simulink model "SS_task9_2021"  (R2021b)
settings: Solver=FixedStepAuto  StartTime=0.0  StopTime=20  FixedStep=0.01  RelTol=1e-3
values from neighbouring files (symbols this model uses):
  A_ss_2dof_vh = eval(subs(A_ss_2dof_vh_sym,{c1,c2},[c,c]))    [Copy_of_Lab_3_ale.m]    (also in SS_task9.m = [0 1 0 0; out8_2.mat = [0 -54.5454545455 0 0 1 -3.63636363636 0 0 0 0 0 -61.7142857; out9.mat = [0 -54.5454545455 0 0 1 0 0 0 0 0 0 -61.7142857143 ... (16 e; vehicle_control.m = [0  1 0 0)
  B_ss_2dof_vh = eval(subs(B_ss_2dof_vh_sym,{c1,c2},[c,c]))    [Copy_of_Lab_3_ale.m]    (also in SS_task9.m = [0 0 0 0; out8_2.mat = [0 27.2727272727 0 -163.636363636 0 1.81818181818 0 -0.34285; out9.mat = [0 27.2727272727 0 -5.14285714286 0 27.2727272727 0 5.142857; vehicle_control.m = [0 0 0 0)
  C_ss_2dof_vh = [1 0 0 0 ... (first row only)    [Copy_of_Lab_3_ale.m]    (also in SS_task9.m = [0 1 0 0; out8_2.mat = [1  0  0  0; 0  0  1  0]; out9.mat = [0  1  0  0; 0  0  0  1]; vehicle_control.m)
  cx = 20e5    (= 2000000)    [SS_task9.m]    (also in out9.mat = 700000)
  cz = 80e3    (= 80000)    [SS_task9.m]    (also in out9.mat = 250000; vehicle_control.m = 150000)
  D_ss_2dof_vh = [0 0 0 0; 0 0 0 0]    [Copy_of_Lab_3_ale.m]    (also in SS_task9.m = [0 0 0 0; out8_2.mat = [0  0  0  0; 0  0  0  0]; out9.mat = [0  0  0  0; 0  0  0  0]; vehicle_control.m)
  L = 6    [Copy_of_Lab_3_ale.m]    (also in H_inf_ctrl.m; H_inf_ctrl_11_2.m; H_inf_ctrl_11_2_m.m; SS_task9.m)
undefined symbols (not defined in the file or in its folder): sigbuilder_block
settings Model: Creator=tawsiful  LastModifiedBy=rivaa
settings DebuggingCC: UnconnectedInputMsg=none  UnconnectedOutputMsg=none  UnconnectedLineMsg=none
settings RTWCC: DLArmComputeVersion=20.02.1

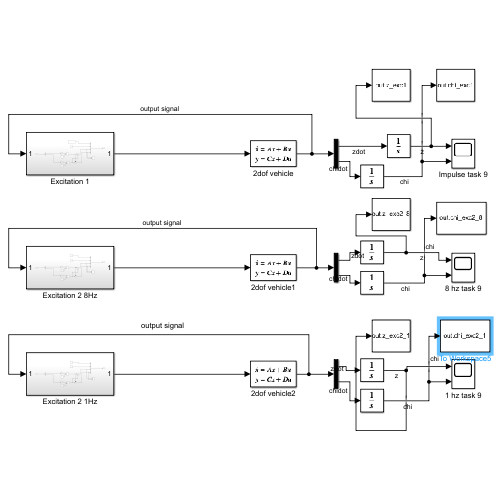
[thumbnail: Simulink's stored preview of the top-level diagram]
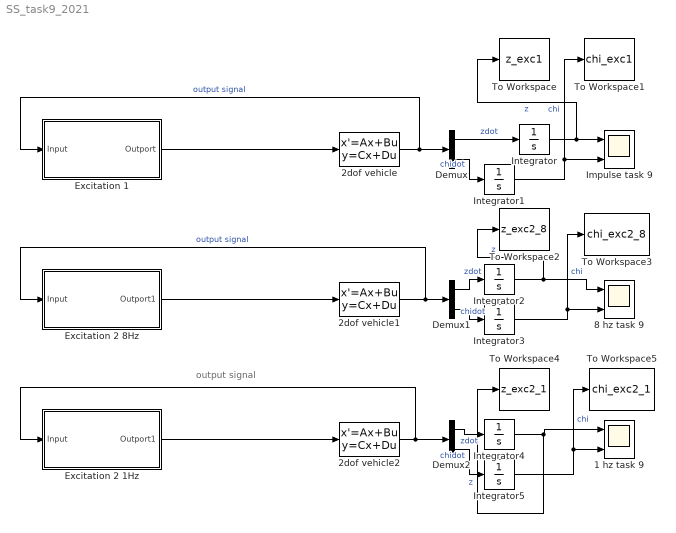
== system SS_task9_2021 ==
  note: output signal
  1 hz task 9 : Scope  NumInputPorts=2
  2dof vehicle : StateSpace  A=A_ss_2dof_vh  B=B_ss_2dof_vh  C=C_ss_2dof_vh  D=D_ss_2dof_vh  InitialCondition=0
  2dof vehicle1 : StateSpace  A=A_ss_2dof_vh  B=B_ss_2dof_vh  C=C_ss_2dof_vh  D=D_ss_2dof_vh  InitialCondition=0
  2dof vehicle2 : StateSpace  A=A_ss_2dof_vh  B=B_ss_2dof_vh  C=C_ss_2dof_vh  D=D_ss_2dof_vh  InitialCondition=0
  8 hz task 9 : Scope  NumInputPorts=2
  Demux : Demux  Outputs=2
  Demux1 : Demux  Outputs=2
  Demux2 : Demux  Outputs=2
  Excitation 1 : Subsystem
  Excitation 2 1Hz : Subsystem
  Excitation 2 8Hz : Subsystem
  Impulse task 9 : Scope  NumInputPorts=2
  Integrator{,1..5} (6 alike) : Integrator
  To Workspace : ToWorkspace  VariableName=z_exc1  SampleTime=-1
      settings: Save2DSignal=2-D array (concatenate along first dimension)
  To Workspace1 : ToWorkspace  VariableName=chi_exc1  SampleTime=-1
      settings: Save2DSignal=2-D array (concatenate along first dimension)
  To Workspace2 : ToWorkspace  VariableName=z_exc2_8  SampleTime=-1
      settings: Save2DSignal=2-D array (concatenate along first dimension)
  To Workspace3 : ToWorkspace  VariableName=chi_exc2_8  SampleTime=-1
      settings: Save2DSignal=2-D array (concatenate along first dimension)
  To Workspace4 : ToWorkspace  VariableName=z_exc2_1  SampleTime=-1
      settings: Save2DSignal=2-D array (concatenate along first dimension)
  To Workspace5 : ToWorkspace  VariableName=chi_exc2_1  SampleTime=-1
      settings: Save2DSignal=2-D array (concatenate along first dimension)
  wires:
  2dof vehicle2/1 -> Excitation 2 1Hz/1(Input), Demux2/1
  Demux2/2 -> Integrator5/1  "chidot"
  Demux1/1 -> Integrator2/1  "zdot"
  Demux2/1 -> Integrator4/1  "zdot"
  Demux/2 -> Integrator1/1  "chidot"
  Demux/1 -> Integrator/1  "zdot"
  Excitation 1/1(Outport) -> 2dof vehicle/1
  2dof vehicle1/1 -> Excitation 2 8Hz/1(Input), Demux1/1  "output signal"
  Demux1/2 -> Integrator3/1  "chidot"
  Excitation 2 8Hz/1(Outport1) -> 2dof vehicle1/1
  2dof vehicle/1 -> Excitation 1/1(Input), Demux/1  "output signal"
  Excitation 2 1Hz/1(Outport1) -> 2dof vehicle2/1
  Integrator/1 -> To Workspace/1, Impulse task 9/1  "z"
  Integrator1/1 -> To Workspace1/1, Impulse task 9/2  "chi"
  Integrator2/1 -> To Workspace2/1, 8 hz task 9/1  "z"
  Integrator3/1 -> To Workspace3/1, 8 hz task 9/2  "chi"
  Integrator4/1 -> To Workspace4/1, 1 hz task 9/1  "z"
  Integrator5/1 -> To Workspace5/1, 1 hz task 9/2  "chi"

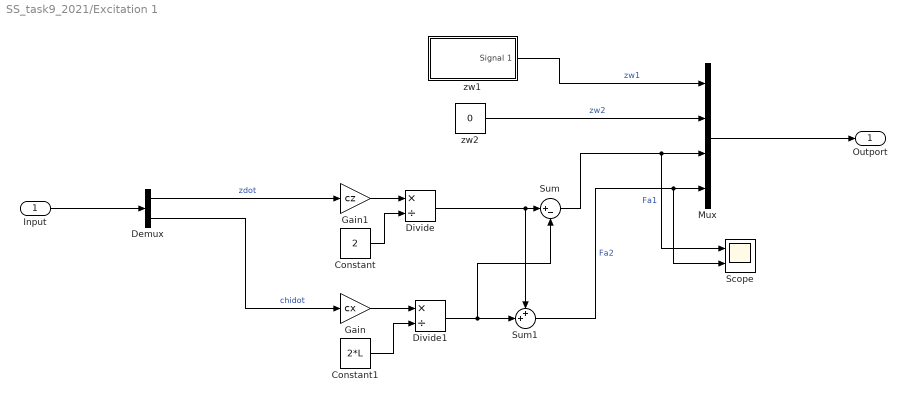
== system SS_task9_2021/Excitation 1 ==
  Input : Inport
  Constant : Constant  Value=2
  Constant1 : Constant  Value=2*L
  Demux : Demux  Outputs=2
  Divide : Product  Inputs=*/
  Divide1 : Product  Inputs=*/
  Gain : Gain  Gain=cx
  Gain1 : Gain  Gain=cz
  Mux : Mux
  Scope : Scope  NumInputPorts=2
  Sum : Sum  Inputs=|+-
  Sum1 : Sum  Inputs=++|
  zw1 : Subsystem  Tag=STV Subsys  LoadFcn=sigbuilder_block('load');  StartFcn=sigbuilder_block('start');  StopFcn=sigbuilder_block('stop');  ClipboardFcn=sigbuilder_block('clipboard');  mask(Sigbuilder block){tuvar=[0:10]}
      mask help: Simulink:masks:SigbuilderBlock_MD
      mask init:
      | if ~strcmp(get_param(bdroot(gcbh),'SimulationStatus'),'stopped') tuvar = sigbuilder_block('maskInit'); end
      settings: CopyFcn=sigbuilder_block('copy');  DeleteFcn=sigbuilder_block('delete');  ModelCloseFcn=sigbuilder_block('modelClose');  PreSaveFcn=sigbuilder_block('preSave');  PauseFcn=sigbuilder_block('pause');  ContinueFcn=sigbuilder_block('continue');  NameChangeFcn=sigbuilder_block('namechange');  OpenFcn=sigbuilder_block('open',[437.6 199.2 550.4 400 ]);  CloseFcn=sigbuilder_block('close');
      mask Display: plot(0, 0, 100, 100,[2, 2, 32, 32, 2], [68, 8, 8, 68, 68],[32, 2], [38, 38], [32, 19, 2],[53, 60, 44], [32, 17, 17, 2],[16, 16, 31, 31]);txt = getActiveGroup(gcbh);text(2, 100, txt,'verticalAlignment', 'top');
  zw2 : Constant  Value=0
  Outport : Outport
  wires:
  zw1/1(Signal 1) -> Mux/1  "zw1"
  Mux/1 -> Outport/1
  zw2/1 -> Mux/2  "zw2"
  Divide/1 -> Sum1/1, Sum/1
  Sum1/1 -> Scope/2, Mux/4  "Fa2"
  Gain1/1 -> Divide/1
  Sum/1 -> Scope/1, Mux/3  "Fa1"
  Divide1/1 -> Sum/2, Sum1/2
  Constant1/1 -> Divide1/2
  Gain/1 -> Divide1/1
  Constant/1 -> Divide/2
  Demux/1 -> Gain1/1  "zdot"
  Demux/2 -> Gain/1  "chidot"
  Input/1 -> Demux/1

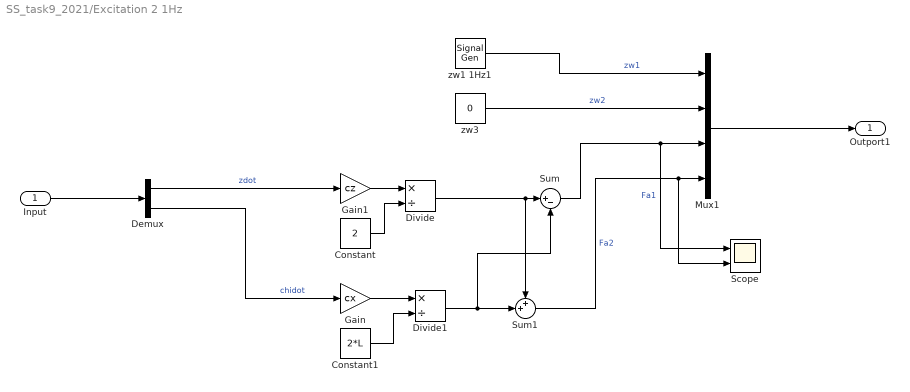
== system SS_task9_2021/Excitation 2 1Hz ==
  Input : Inport
  Constant : Constant  Value=2
  Constant1 : Constant  Value=2*L
  Demux : Demux  Outputs=2
  Divide : Product  Inputs=*/
  Divide1 : Product  Inputs=*/
  Gain : Gain  Gain=cx
  Gain1 : Gain  Gain=cz
  Mux1 : Mux
  Scope : Scope  NumInputPorts=2
  Sum : Sum  Inputs=|+-
  Sum1 : Sum  Inputs=++|
  zw1 1Hz1 : SignalGenerator  Amplitude=0.01  Frequency=2*pi*1  Units=rad/sec
  zw3 : Constant  Value=0
  Outport1 : Outport
  wires:
  Demux/2 -> Gain/1  "chidot"
  Input/1 -> Demux/1
  Gain1/1 -> Divide/1
  zw3/1 -> Mux1/2  "zw2"
  Mux1/1 -> Outport1/1
  zw1 1Hz1/1 -> Mux1/1  "zw1"
  Constant/1 -> Divide/2
  Divide1/1 -> Sum/2, Sum1/2
  Gain/1 -> Divide1/1
  Divide/1 -> Sum1/1, Sum/1
  Constant1/1 -> Divide1/2
  Demux/1 -> Gain1/1  "zdot"
  Sum1/1 -> Scope/2, Mux1/4  "Fa2"
  Sum/1 -> Scope/1, Mux1/3  "Fa1"

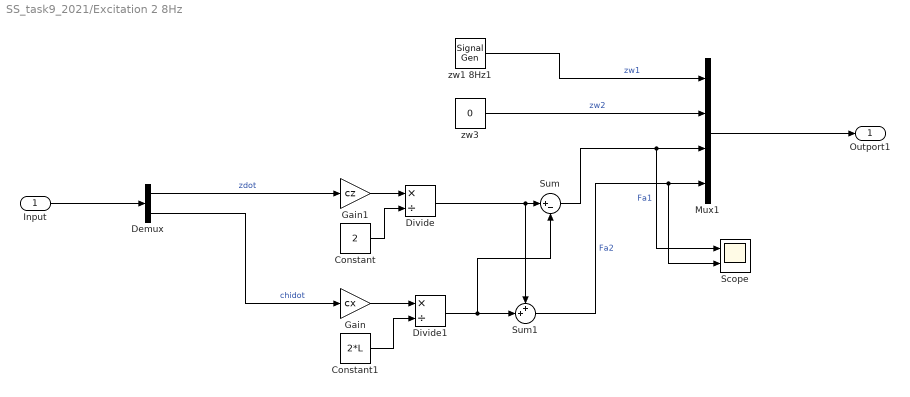
== system SS_task9_2021/Excitation 2 8Hz ==
  Input : Inport
  Constant : Constant  Value=2
  Constant1 : Constant  Value=2*L
  Demux : Demux  Outputs=2
  Divide : Product  Inputs=*/
  Divide1 : Product  Inputs=*/
  Gain : Gain  Gain=cx
  Gain1 : Gain  Gain=cz
  Mux1 : Mux
  Scope : Scope  NumInputPorts=2
  Sum : Sum  Inputs=|+-
  Sum1 : Sum  Inputs=++|
  zw1 8Hz1 : SignalGenerator  Amplitude=0.01  Frequency=2*pi*8  Units=rad/sec
  zw3 : Constant  Value=0
  Outport1 : Outport
  wires:
  Demux/2 -> Gain/1  "chidot"
  Input/1 -> Demux/1
  Gain1/1 -> Divide/1
  zw3/1 -> Mux1/2  "zw2"
  Mux1/1 -> Outport1/1
  zw1 8Hz1/1 -> Mux1/1  "zw1"
  Constant/1 -> Divide/2
  Divide1/1 -> Sum/2, Sum1/2
  Gain/1 -> Divide1/1
  Divide/1 -> Sum1/1, Sum/1
  Constant1/1 -> Divide1/2
  Demux/1 -> Gain1/1  "zdot"
  Sum1/1 -> Scope/2, Mux1/4  "Fa2"
  Sum/1 -> Scope/1, Mux1/3  "Fa1"

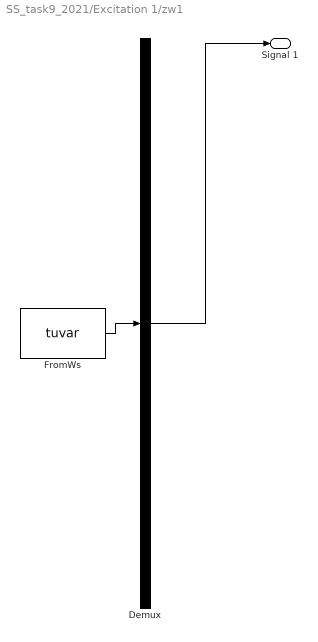
== system SS_task9_2021/Excitation 1/zw1 ==
  Demux : Demux  Tag=STV Demux  Outputs=1
      settings: DisplayOption=none
  FromWs : FromWorkspace  Tag=STV FromWs  VariableName=tuvar
      SigBuilderData=|
      | common.afterFinalStr = 'Extrapolate'
      | common.sampleTime = 0
      | dataSet.timeRange = [0 10]
      | dataSet.name = 'Group 1'
      | sbobj.Groups.Name = 'Group 1'
      | sbobj.Groups.Signals.Name = 'Signal 1'
      | sbobj.Groups.Signals.XData = [0 0.1 0.1 10]
      | sbobj.Groups.Signals.YData = [0.03 0.03 0 0]
  Signal 1 : Outport  Tag=STV Outport
  wires:
  Demux/1 -> Signal 1/1
  FromWs/1 -> Demux/1
